simulink model "vtol_lon_no_ctrl"  (R2024b)
settings: Solver=VariableStepAuto  StartTime=0.0  StopTime=10.0  RelTol=1e-3
undefined symbols (not defined in the file or in its folder): A_vtol_lon, B_vtol_lon, C_vtol_lon, D_vtol_lon
settings Model: Creator=mhcho  LastModifiedBy=mhcho

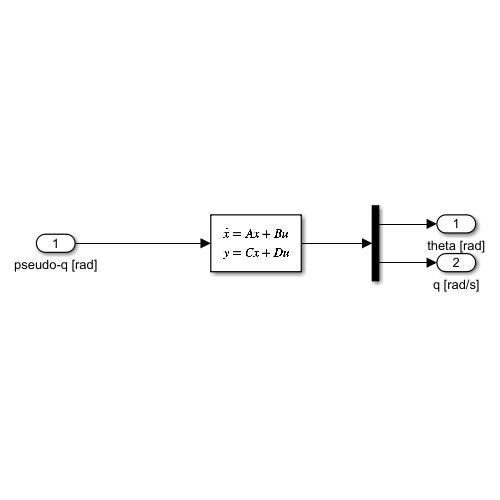
[thumbnail: Simulink's stored preview of the top-level diagram]
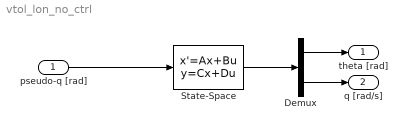
== system vtol_lon_no_ctrl ==
  pseudo-q [rad] : Inport
  Demux : Demux  Outputs=2
  State-Space : StateSpace  A=A_vtol_lon(3:4,3:4)  B=B_vtol_lon(3:4,1)  C=C_vtol_lon(3:4,3:4)  D=D_vtol_lon(3:4,1)  InitialCondition=0
  theta [rad] : Outport
  q [rad/s] : Outport  Port=2
  wires:
  pseudo-q [rad]/1 -> State-Space/1
  State-Space/1 -> Demux/1
  Demux/1 -> theta [rad]/1
  Demux/2 -> q [rad/s]/1
